simulink model "q2_model"  (R2016a)
settings: Solver=VariableStepAuto  StartTime=0.0  StopTime=40  RelTol=1e-3
values from neighbouring files (symbols this model uses):
  A = [0 1  0              0 ... (first row only)    [MatLab4p.m]    (also in MatLab5p.m = [     0        1       0        0; MatLab6p.m = [     0        1       0        0; _Labs.m = [     0        1       0        0; q2.m = [0 1  0   0)
  Am = blkdiag(M,M)    [MatLab5p.m]    (also in MatLab6p.m; _Labs.m; q2.m = 1; questao2.m = 1)
  B = [0; 1/M; 0; -1/(M*L)]    [MatLab4p.m]    (also in MatLab5p.m = [ 0    0; MatLab6p.m = [ 0    0; _Labs.m = [ 0    0; q2.m = [  0)
  Bm = blkdiag(N,N)    [MatLab5p.m]    (also in MatLab6p.m; _Labs.m; q2.m = N; questao2.m = N)
  C = [1 0 0 0]    [MatLab4p.m]    (also in MatLab5p.m = [1 0 0 0; MatLab6p.m = [1 0 0 0; _Labs.m = [1 0 0 0; q2.m)
  Cm = eye(1)    [q2.m]    (also in questao2.m = eye(3))
  Dm = zeros(1,1)    [q2.m]    (also in questao2.m = zeros(3,1))
  Dsim = zeros(4,1)    [MatLab4p.m]    (also in MatLab5p.m = zeros(4,2); MatLab6p.m = zeros(4,2); _Labs.m = zeros(4,2); q2.m)
  K = place(A,B,[-2 -2.05 -2.1 -2.15])    [MatLab4p.m]    (also in MatLab5p.m = Ka(:,1:4); MatLab6p.m = Ka(:,1:4); _Labs.m = Ka(:,1:4); q2.m = Ka(:,1:4))
  Km = Ka(:,5:10)    [MatLab5p.m]    (also in MatLab6p.m; _Labs.m; q2.m = Ka(5); questao2.m = Ka(:,5:7))
  x0 = [0 0 pi/4 0]    [MatLab4p.m]    (also in MatLab5p.m = [1 0.5 1 0.1]; MatLab6p.m = [1 2 0.8 -0.3]; _Labs.m = [1 2 0.8 -0.3]; q2.m = [0 0 0 0])
settings Model: Creator=ivan_prog  LastModifiedBy=ivan_prog

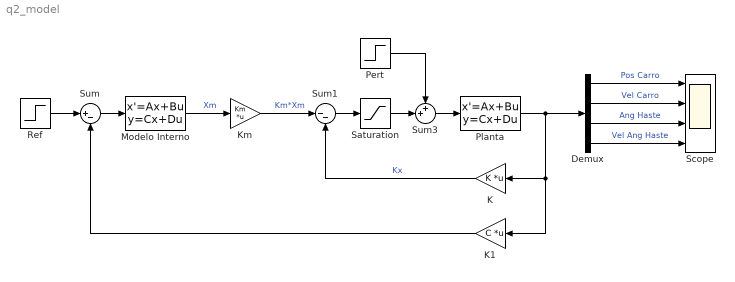
== system q2_model ==
  Demux : Demux
  K : Gain  Gain=K  Multiplication=Matrix(K*u)
  K1 : Gain  Gain=C  Multiplication=Matrix(K*u)
  Km : Gain  Gain=Km  Multiplication=Matrix(K*u)
  Modelo Interno : StateSpace  A=Am  B=Bm  C=Cm  D=Dm  X0=[0]
  Pert : Step  Time=20  After=.8  SampleTime=0
  Planta : StateSpace  A=A  B=B  C=eye(4)  D=Dsim  X0=x0
  Ref : Step  Time=0  SampleTime=0
  Saturation : Saturate  UpperLimit=50  LowerLimit=-50
  Scope : Scope  NumInputPorts=4
  Sum : Sum  Inputs=|+-
  Sum1 : Sum  Inputs=|--
  Sum3 : Sum  Inputs=++|
  wires:
  Planta/1 -> Demux/1, K1/1, K/1
  Ref/1 -> Sum/1
  Sum/1 -> Modelo Interno/1
  Km/1 -> Sum1/1  "Km*Xm"
  K/1 -> Sum1/2  "Kx"
  Sum3/1 -> Planta/1
  Pert/1 -> Sum3/1
  Modelo Interno/1 -> Km/1  "Xm"
  Sum1/1 -> Saturation/1
  Saturation/1 -> Sum3/2
  K1/1 -> Sum/2
  Demux/1 -> Scope/1  "Pos Carro"
  Demux/2 -> Scope/2  "Vel Carro"
  Demux/3 -> Scope/3  "Ang Haste"
  Demux/4 -> Scope/4  "Vel Ang Haste"
